simulink model "plantFunction_harness"  (R2024a)
settings: Solver=VariableStepAuto  StartTime=0.0  StopTime=10.0  RelTol=1e-3
settings Model: Creator=tn212  LastModifiedBy=tn212

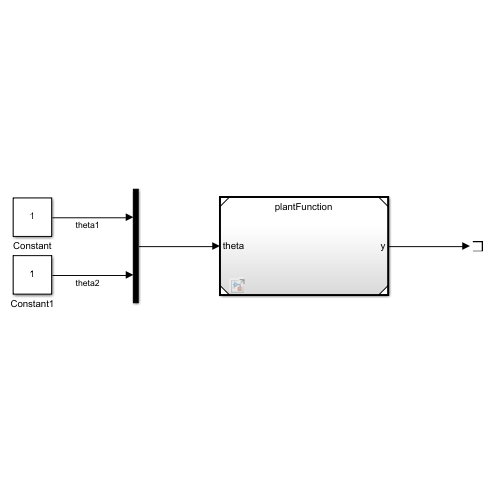
[thumbnail: Simulink's stored preview of the top-level diagram]
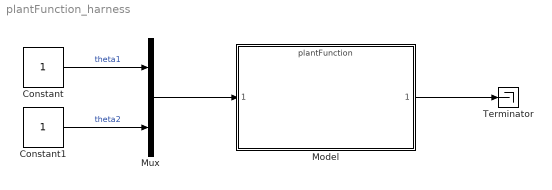
== system plantFunction_harness ==
  Constant : Constant  VectorParams1D=off  SampleTime=-1
  Constant1 : Constant  VectorParams1D=off  SampleTime=-1
  Model : ModelReference  ModelNameDialog=plantFunction.slx  SimulationMode=Normal  ModelReferenceVersion=1.4
  Mux : Mux  Inputs=2
  Terminator : Terminator
  wires:
  Mux/1 -> Model/1
  Model/1 -> Terminator/1
  Constant/1 -> Mux/1  "theta1"
  Constant1/1 -> Mux/2  "theta2"
